simulink library "rewardLibrary"  (R2022b)
settings: Solver=VariableStepAuto  StartTime=0.0  StopTime=10.0  RelTol=1e-3
values from neighbouring files (symbols this model uses):
  accel_vec = (-4:0.5:4)'    [setUpModel.m]
  Ts = 0.1    [setUpMPC.m]
  TsRL = Ts    [setUpRLEnv.m]
  vel_vec = 0:2:20    [setUpModel.m]
undefined symbols (not defined in the file or in its folder): A, B, C, curvature1, D, D_default, DiscIntNeverNeededParam, E, F, gradbp1, k_sigmoid, steer_lim, t_gap, v_set, x_colpen, y_colpen, Z_colpen
libraries: simulink x379, $bdroot x2, mpcadaslib x1
(part 5 of 9)

== system rewardLibrary/Obs // Reward 3-6/Subsystem1 ==
  steer : Inport
  e1 : Inport  Port=2
  v_err : Inport  Port=3
  accel : Inport  Port=4
  Compare To Constant : simulink/Logic and Bit Operations/Compare To Constant  relop=<  const=1  OutDataTypeStr=boolean
  Compare To Constant1 : simulink/Logic and Bit Operations/Compare To Constant  relop=<  const=16  OutDataTypeStr=boolean
  Constant2 : Constant  Value=0
  Constant3 : Constant  Value=5
  Digital Clock : DigitalClock  SampleTime=Ts
  Gain1 : Gain
  Gain2 : Gain  Gain=500
  Gain3 : Gain  Gain=2
  Gain4 : Gain  Gain=1e-3
  Gain6 : Gain  Gain=100
  Gain7 : Gain  Gain=15
  Gain8 : Gain  Gain=100
  Math Function2 : Math  Operator=square  SignedPower=on
  Square : Math  Operator=square  SignedPower=on
  Square2 : Math  Operator=square  SignedPower=on
  Square5 : Math  Operator=square  SignedPower=on
  Sum : Sum  Inputs=-----
  Sum1 : Sum  Inputs=++++
  Switch2 : Switch  Criteria=u2 > Threshold  Threshold=10  SaturateOnIntegerOverflow=off  InputSameDT=off
  Unit Delay : UnitDelay  SampleTime=-1  HasFrameUpgradeWarning=on
  Unit Delay1 : UnitDelay  SampleTime=-1  HasFrameUpgradeWarning=on
  turn assist : Subsystem  Commented=on
  reward : Outport  VectorParamsAs1DForOutWhenUnconnected=off
  wires:
  v_err/1 -> Square5/1
  Square/1 -> Compare To Constant1/1, Gain8/1
  Sum1/1 -> reward/1
  accel/1 -> Unit Delay1/1
  Gain6/1 -> Sum/5
  Compare To Constant/1 -> Gain1/1
  Math Function2/1 -> Gain6/1
  Gain3/1 -> Sum1/1
  Compare To Constant1/1 -> Gain3/1
  Square2/1 -> Gain2/1
  Gain7/1 -> Sum/4
  Unit Delay1/1 -> Math Function2/1
  Gain1/1 -> Sum1/3
  steer/1 -> Unit Delay/1
  Gain2/1 -> Sum/3
  Sum/1 -> Gain4/1
  Unit Delay/1 -> turn assist/1(u_prev), Square2/1  "u_prev"
  Square5/1 -> Compare To Constant/1, Gain7/1
  Gain4/1 -> Sum1/2
  e1/1 -> Square/1
  Digital Clock/1 -> Switch2/2
  Switch2/1 -> Sum1/4
  Gain8/1 -> Sum/1
  Constant2/1 -> Switch2/3
  Constant3/1 -> Switch2/1
  turn assist/1(Out1) -> Sum/2

== system rewardLibrary/Obs // Reward 3-6/Subsystem2 ==
  v_ego : Inport
  e1 : Inport  Port=2
  e2 : Inport  Port=3
  AND : Logic  IconShape=distinctive  AllPortsSameDT=off  OutDataTypeStr=boolean
  Abs : Abs  SaturateOnIntegerOverflow=off
  Abs1 : Abs  SaturateOnIntegerOverflow=off
  Lateral deviation : simulink/Logic and Bit Operations/Compare To Constant  relop=>  const=12  OutDataTypeStr=boolean
  Logical Operator1 : Logic  Operator=OR  AllPortsSameDT=off  OutDataTypeStr=boolean
  R2D : Gain  Gain=180/pi
  Relative yaw angle : simulink/Logic and Bit Operations/Compare To Constant  relop=>  const=55  OutDataTypeStr=boolean
  Velocity : simulink/Logic and Bit Operations/Compare To Constant  relop=<  const=2  OutDataTypeStr=boolean
  Velocity1 : simulink/Logic and Bit Operations/Compare To Constant  relop=<  const=5  OutDataTypeStr=boolean
  offTrack : Outport  VectorParamsAs1DForOutWhenUnconnected=off
  tooSlow / spinTurn : Outport  Port=2  VectorParamsAs1DForOutWhenUnconnected=off
  wires:
  Velocity/1 -> Logical Operator1/1  "tooSlow"
  Lateral deviation/1 -> offTrack/1
  v_ego/1 -> Velocity1/1, Velocity/1
  Abs/1 -> Lateral deviation/1
  e1/1 -> Abs/1
  Velocity1/1 -> AND/1
  e2/1 -> Abs1/1
  Abs1/1 -> R2D/1
  R2D/1 -> Relative yaw angle/1
  Relative yaw angle/1 -> AND/2
  AND/1 -> Logical Operator1/2  "spinTurn"
  Logical Operator1/1 -> tooSlow / spinTurn/1

== system rewardLibrary/Obs // Reward 4-1/Subsystem ==
  v_ego : Inport
  v_ref : Inport  Port=2
  e1 : Inport  Port=3
  e2 : Inport  Port=4
  e1dot : Inport  Port=5
  e2dot : Inport  Port=6
  Add : Sum  Inputs=+-
  Discrete-Time Integrator1 : DiscreteIntegrator  SampleTime=-1  ICPrevOutput=DiscIntNeverNeededParam  ICPrevScaledInput=DiscIntNeverNeededParam
  Discrete-Time Integrator2 : DiscreteIntegrator  SampleTime=-1  ICPrevOutput=DiscIntNeverNeededParam  ICPrevScaledInput=DiscIntNeverNeededParam
  Discrete-Time Integrator3 : DiscreteIntegrator  SampleTime=-1  ICPrevOutput=DiscIntNeverNeededParam  ICPrevScaledInput=DiscIntNeverNeededParam
  Lateral deviation : Scope
  Mux : Mux  Inputs=9
  obs : Outport  VectorParamsAs1DForOutWhenUnconnected=off
  v_err : Outport  Port=2  VectorParamsAs1DForOutWhenUnconnected=off
  wires:
  Add/1 -> v_err/1, Mux/2, Discrete-Time Integrator1/1
  Discrete-Time Integrator3/1 -> Mux/6  "integral_error"
  v_ego/1 -> Add/2, Mux/3
  e1/1 -> Lateral deviation/1, Mux/5, Discrete-Time Integrator2/1
  Discrete-Time Integrator1/1 -> Mux/1  "integral_error"
  e2/1 -> Mux/7, Discrete-Time Integrator3/1
  Discrete-Time Integrator2/1 -> Mux/4  "integral_error"
  Mux/1 -> obs/1
  e1dot/1 -> Mux/8
  e2dot/1 -> Mux/9
  v_ref/1 -> Add/1  "d_rel"

== system rewardLibrary/Obs // Reward 4-1/Subsystem1 ==
  steer : Inport
  e1 : Inport  Port=2
  v_err : Inport  Port=3
  accel : Inport  Port=4
  Compare To Constant : simulink/Logic and Bit Operations/Compare To Constant  relop=<  const=1  OutDataTypeStr=boolean
  Compare To Constant1 : simulink/Logic and Bit Operations/Compare To Constant  relop=<  const=16  OutDataTypeStr=boolean
  Compare To Constant2 : simulink/Logic and Bit Operations/Compare To Constant  relop=>  const=-20  OutDataTypeStr=boolean
  Constant : Constant  Value=1000
  Constant1 : Constant  Value=0
  Demux : Demux  Outputs=2
  Detect Rise Positive : simulink/Logic and Bit Operations/Detect Rise Positive  vinit=0  OutDataTypeStr=boolean
  Gain1 : Gain
  Gain2 : Gain  Gain=500
  Gain3 : Gain  Gain=2
  Gain4 : Gain  Gain=1e-3
  Gain6 : Gain  Gain=100
  Gain7 : Gain  Gain=20
  Gain8 : Gain  Gain=100
  Math Function2 : Math  Operator=square  SignedPower=on
  Square : Math  Operator=square  SignedPower=on
  Square2 : Math  Operator=square  SignedPower=on
  Square5 : Math  Operator=square  SignedPower=on
  Sum : Sum  Inputs=-----
  Sum1 : Sum  Inputs=++++
  Switch : Switch  Criteria=u2 > Threshold  SaturateOnIntegerOverflow=off  InputSameDT=off
  Terminator : Terminator
  Unit Delay : UnitDelay  SampleTime=-1  HasFrameUpgradeWarning=on
  Unit Delay1 : UnitDelay  SampleTime=-1  HasFrameUpgradeWarning=on
  time reward : Subsystem  Commented=on
  turn assist : Subsystem  Commented=on
  reward : Outport  VectorParamsAs1DForOutWhenUnconnected=off
  wires:
  v_err/1 -> Square5/1
  Square/1 -> Compare To Constant1/1, Gain8/1
  Sum1/1 -> reward/1
  accel/1 -> Unit Delay1/1
  Gain6/1 -> Sum/5
  Compare To Constant/1 -> Gain1/1
  Math Function2/1 -> Gain6/1
  Gain3/1 -> Sum1/1
  Compare To Constant1/1 -> Gain3/1
  Square2/1 -> Gain2/1
  Gain7/1 -> Sum/4
  Unit Delay1/1 -> Math Function2/1
  Gain1/1 -> Sum1/3
  steer/1 -> Unit Delay/1
  Gain2/1 -> Sum/3
  Sum/1 -> Gain4/1
  Unit Delay/1 -> turn assist/1(u_prev), Square2/1  "u_prev"
  Square5/1 -> Compare To Constant/1, Gain7/1
  Gain4/1 -> Sum1/2
  e1/1 -> Square/1
  Gain8/1 -> Sum/1
  turn assist/1(Out1) -> Sum/2
  [pos2] -> Demux/1
  Demux/1 -> Terminator/1
  Demux/2 -> Compare To Constant2/1  "y2"
  Constant/1 -> Switch/1
  Constant1/1 -> Switch/3
  Compare To Constant2/1 -> Detect Rise Positive/1
  Detect Rise Positive/1 -> Switch/2
  Switch/1 -> Sum1/4  "madeCorner"

== system rewardLibrary/Obs // Reward 4-1/Subsystem2 ==
  v_ego : Inport
  e1 : Inport  Port=2
  e2 : Inport  Port=3
  AND : Logic  IconShape=distinctive  AllPortsSameDT=off  OutDataTypeStr=boolean
  Abs : Abs  SaturateOnIntegerOverflow=off
  Abs1 : Abs  SaturateOnIntegerOverflow=off
  Lateral deviation : simulink/Logic and Bit Operations/Compare To Constant  relop=>  const=12  OutDataTypeStr=boolean
  Logical Operator1 : Logic  Operator=OR  AllPortsSameDT=off  OutDataTypeStr=boolean
  R2D : Gain  Gain=180/pi
  Relative yaw angle : simulink/Logic and Bit Operations/Compare To Constant  relop=>  const=55  OutDataTypeStr=boolean
  Velocity : simulink/Logic and Bit Operations/Compare To Constant  relop=<  const=2  OutDataTypeStr=boolean
  Velocity1 : simulink/Logic and Bit Operations/Compare To Constant  relop=<  const=5  OutDataTypeStr=boolean
  offTrack : Outport  VectorParamsAs1DForOutWhenUnconnected=off
  tooSlow / spinTurn : Outport  Port=2  VectorParamsAs1DForOutWhenUnconnected=off
  wires:
  Velocity/1 -> Logical Operator1/1  "tooSlow"
  Lateral deviation/1 -> offTrack/1
  v_ego/1 -> Velocity1/1, Velocity/1
  Abs/1 -> Lateral deviation/1
  e1/1 -> Abs/1
  Velocity1/1 -> AND/1
  e2/1 -> Abs1/1
  Abs1/1 -> R2D/1
  R2D/1 -> Relative yaw angle/1
  Relative yaw angle/1 -> AND/2
  AND/1 -> Logical Operator1/2  "spinTurn"
  Logical Operator1/1 -> tooSlow / spinTurn/1

== system rewardLibrary/Obs // Reward 4-2/Subsystem ==
  v_ego : Inport
  v_ref : Inport  Port=2
  e1 : Inport  Port=3
  e2 : Inport  Port=4
  e1dot : Inport  Port=5
  e2dot : Inport  Port=6
  Add : Sum  Inputs=+-
  Discrete-Time Integrator1 : DiscreteIntegrator  SampleTime=-1  ICPrevOutput=DiscIntNeverNeededParam  ICPrevScaledInput=DiscIntNeverNeededParam
  Discrete-Time Integrator2 : DiscreteIntegrator  SampleTime=-1  ICPrevOutput=DiscIntNeverNeededParam  ICPrevScaledInput=DiscIntNeverNeededParam
  Discrete-Time Integrator3 : DiscreteIntegrator  SampleTime=-1  ICPrevOutput=DiscIntNeverNeededParam  ICPrevScaledInput=DiscIntNeverNeededParam
  Lateral deviation : Scope
  Mux : Mux  Inputs=9
  obs : Outport  VectorParamsAs1DForOutWhenUnconnected=off
  v_err : Outport  Port=2  VectorParamsAs1DForOutWhenUnconnected=off
  wires:
  Add/1 -> v_err/1, Mux/2, Discrete-Time Integrator1/1
  Discrete-Time Integrator3/1 -> Mux/6  "integral_error"
  v_ego/1 -> Add/2, Mux/3
  e1/1 -> Lateral deviation/1, Mux/5, Discrete-Time Integrator2/1
  Discrete-Time Integrator1/1 -> Mux/1  "integral_error"
  e2/1 -> Mux/7, Discrete-Time Integrator3/1
  Discrete-Time Integrator2/1 -> Mux/4  "integral_error"
  Mux/1 -> obs/1
  e1dot/1 -> Mux/8
  e2dot/1 -> Mux/9
  v_ref/1 -> Add/1  "d_rel"

== system rewardLibrary/Obs // Reward 4-2/Subsystem1 ==
  steer : Inport
  e1 : Inport  Port=2
  v_err : Inport  Port=3
  accel : Inport  Port=4
  Compare To Constant : simulink/Logic and Bit Operations/Compare To Constant  relop=<  const=1  OutDataTypeStr=boolean
  Compare To Constant1 : simulink/Logic and Bit Operations/Compare To Constant  relop=<  const=16  OutDataTypeStr=boolean
  Compare To Constant2 : simulink/Logic and Bit Operations/Compare To Constant  relop=>  const=-20  OutDataTypeStr=boolean
  Constant : Constant  Value=1000
  Constant1 : Constant  Value=0
  Demux : Demux  Outputs=2
  Detect Rise Positive : simulink/Logic and Bit Operations/Detect Rise Positive  vinit=0  OutDataTypeStr=boolean
  Gain1 : Gain
  Gain2 : Gain  Gain=500
  Gain3 : Gain  Gain=2
  Gain4 : Gain  Gain=1e-3
  Gain6 : Gain  Gain=100
  Gain7 : Gain  Gain=20
  Gain8 : Gain  Gain=100
  Math Function2 : Math  Operator=square  SignedPower=on
  Square : Math  Operator=square  SignedPower=on
  Square2 : Math  Operator=square  SignedPower=on
  Square5 : Math  Operator=square  SignedPower=on
  Sum : Sum  Inputs=-----
  Sum1 : Sum  Inputs=++++
  Switch : Switch  Criteria=u2 > Threshold  SaturateOnIntegerOverflow=off  InputSameDT=off
  Terminator : Terminator
  Unit Delay : UnitDelay  SampleTime=-1  HasFrameUpgradeWarning=on
  Unit Delay1 : UnitDelay  SampleTime=-1  HasFrameUpgradeWarning=on
  time reward : Subsystem  Commented=on
  turn assist : Subsystem  Commented=on
  reward : Outport  VectorParamsAs1DForOutWhenUnconnected=off
  wires:
  v_err/1 -> Square5/1
  Square/1 -> Compare To Constant1/1, Gain8/1
  Sum1/1 -> reward/1
  accel/1 -> Unit Delay1/1
  Gain6/1 -> Sum/5
  Compare To Constant/1 -> Gain1/1
  Math Function2/1 -> Gain6/1
  Gain3/1 -> Sum1/1
  Compare To Constant1/1 -> Gain3/1
  Square2/1 -> Gain2/1
  Gain7/1 -> Sum/4
  Unit Delay1/1 -> Math Function2/1
  Gain1/1 -> Sum1/3
  steer/1 -> Unit Delay/1
  Gain2/1 -> Sum/3
  Sum/1 -> Gain4/1
  Unit Delay/1 -> turn assist/1(u_prev), Square2/1  "u_prev"
  Square5/1 -> Compare To Constant/1, Gain7/1
  Gain4/1 -> Sum1/2
  e1/1 -> Square/1
  Gain8/1 -> Sum/1
  turn assist/1(Out1) -> Sum/2
  [pos2] -> Demux/1
  Demux/1 -> Terminator/1
  Demux/2 -> Compare To Constant2/1  "y2"
  Constant/1 -> Switch/1
  Constant1/1 -> Switch/3
  Compare To Constant2/1 -> Detect Rise Positive/1
  Detect Rise Positive/1 -> Switch/2
  Switch/1 -> Sum1/4  "madeCorner"

== system rewardLibrary/Obs // Reward 4-2/Subsystem2 ==
  v_ego : Inport
  e1 : Inport  Port=2
  e2 : Inport  Port=3
  AND : Logic  IconShape=distinctive  AllPortsSameDT=off  OutDataTypeStr=boolean
  Abs : Abs  SaturateOnIntegerOverflow=off
  Abs1 : Abs  SaturateOnIntegerOverflow=off
  Lateral deviation : simulink/Logic and Bit Operations/Compare To Constant  relop=>  const=8  OutDataTypeStr=boolean
  R2D : Gain  Gain=180/pi
  Relative yaw angle : simulink/Logic and Bit Operations/Compare To Constant  relop=>  const=55  OutDataTypeStr=boolean
  Velocity : simulink/Logic and Bit Operations/Compare To Constant  relop=<  const=2  OutDataTypeStr=boolean
  Velocity1 : simulink/Logic and Bit Operations/Compare To Constant  relop=<  const=5  OutDataTypeStr=boolean
  offTrack : Outport  VectorParamsAs1DForOutWhenUnconnected=off
  tooSlow : Outport  Port=2  VectorParamsAs1DForOutWhenUnconnected=off
  spinTurn : Outport  Port=3  VectorParamsAs1DForOutWhenUnconnected=off
  wires:
  Velocity/1 -> tooSlow/1  "tooSlow"
  Lateral deviation/1 -> offTrack/1
  v_ego/1 -> Velocity1/1, Velocity/1
  Abs/1 -> Lateral deviation/1
  e1/1 -> Abs/1
  Velocity1/1 -> AND/1
  e2/1 -> Abs1/1
  Abs1/1 -> R2D/1
  R2D/1 -> Relative yaw angle/1
  Relative yaw angle/1 -> AND/2
  AND/1 -> spinTurn/1  "spinTurn"

== system rewardLibrary/Obs // Reward 5-1/Subsystem ==
  v_ego : Inport
  v_ref : Inport  Port=2
  e1 : Inport  Port=3
  e2 : Inport  Port=4
  e1dot : Inport  Port=5
  e2dot : Inport  Port=6
  Add : Sum  Inputs=+-
  Discrete-Time Integrator1 : DiscreteIntegrator  SampleTime=-1  ICPrevOutput=DiscIntNeverNeededParam  ICPrevScaledInput=DiscIntNeverNeededParam
  Discrete-Time Integrator2 : DiscreteIntegrator  SampleTime=-1  ICPrevOutput=DiscIntNeverNeededParam  ICPrevScaledInput=DiscIntNeverNeededParam
  Discrete-Time Integrator3 : DiscreteIntegrator  SampleTime=-1  ICPrevOutput=DiscIntNeverNeededParam  ICPrevScaledInput=DiscIntNeverNeededParam
  Lateral deviation : Scope
  Mux : Mux  Inputs=9
  obs : Outport  VectorParamsAs1DForOutWhenUnconnected=off
  v_err : Outport  Port=2  VectorParamsAs1DForOutWhenUnconnected=off
  wires:
  Add/1 -> v_err/1, Mux/2, Discrete-Time Integrator1/1
  Discrete-Time Integrator3/1 -> Mux/6  "integral_error"
  v_ego/1 -> Add/2, Mux/3
  e1/1 -> Lateral deviation/1, Mux/5, Discrete-Time Integrator2/1
  Discrete-Time Integrator1/1 -> Mux/1  "integral_error"
  e2/1 -> Mux/7, Discrete-Time Integrator3/1
  Discrete-Time Integrator2/1 -> Mux/4  "integral_error"
  Mux/1 -> obs/1
  e1dot/1 -> Mux/8
  e2dot/1 -> Mux/9
  v_ref/1 -> Add/1  "d_rel"

== system rewardLibrary/Obs // Reward 5-1/Subsystem1 ==
  v_err : Inport
  e1 : Inport  Port=2
  e2 : Inport  Port=3
  steer : Inport  Port=4
  accel : Inport  Port=5
  Exp{,1..4} (5 alike) : Math
  Gain1 : Gain  Gain=0.5
  Gain10 : Gain  Gain=-0.1
  Gain2 : Gain  Gain=0.2
  Gain3 : Gain  Gain=0.1
  Gain4 : Gain  Gain=-0.5
  Gain5 : Gain  Gain=-10
  Gain6 : Gain  Gain=1.5
  Gain7 : Gain
  Gain8 : Gain  Gain=-0.1
  Gain9 : Gain  Gain=-1.5
  Math Function2 : Math  Operator=square  SignedPower=on
  Square{1..3,5} (4 alike) : Math  Operator=square  SignedPower=on
  Sum1 : Sum  Inputs=+++++
  Unit Delay : UnitDelay  SampleTime=-1  HasFrameUpgradeWarning=on
  Unit Delay1 : UnitDelay  SampleTime=-1  HasFrameUpgradeWarning=on
  reward : Outport  VectorParamsAs1DForOutWhenUnconnected=off
  wires:
  Sum1/1 -> reward/1
  accel/1 -> Unit Delay1/1
  Square2/1 -> Gain4/1
  steer/1 -> Unit Delay/1
  Square5/1 -> Gain10/1
  e1/1 -> Square1/1
  v_err/1 -> Square5/1
  e2/1 -> Square2/1
  Unit Delay/1 -> Math Function2/1  "u_prev"
  Unit Delay1/1 -> Square3/1
  Square3/1 -> Gain8/1
  Math Function2/1 -> Gain5/1
  Square1/1 -> Gain9/1
  Gain10/1 -> Exp/1
  Gain8/1 -> Exp4/1
  Gain5/1 -> Exp3/1
  Gain4/1 -> Exp2/1
  Gain9/1 -> Exp1/1
  Exp/1 -> Gain7/1
  Exp1/1 -> Gain6/1
  Exp2/1 -> Gain1/1
  Exp3/1 -> Gain2/1
  Exp4/1 -> Gain3/1
  Gain3/1 -> Sum1/5
  Gain2/1 -> Sum1/4
  Gain1/1 -> Sum1/3
  Gain6/1 -> Sum1/2
  Gain7/1 -> Sum1/1

== system rewardLibrary/Obs // Reward 5-1/Subsystem2 ==
  v_ego : Inport
  e1 : Inport  Port=2
  e2 : Inport  Port=3
  AND : Logic  Commented=on  IconShape=distinctive  AllPortsSameDT=off  OutDataTypeStr=boolean
  Abs : Abs  SaturateOnIntegerOverflow=off
  Abs1 : Abs  Commented=on  SaturateOnIntegerOverflow=off
  Lateral deviation : simulink/Logic and Bit Operations/Compare To Constant  relop=>  const=8  OutDataTypeStr=boolean
  R2D : Gain  Commented=on  Gain=180/pi
  Relative yaw angle : simulink/Logic and Bit Operations/Compare To Constant  Commented=on  relop=>  const=55  OutDataTypeStr=boolean
  Velocity : simulink/Logic and Bit Operations/Compare To Constant  relop=<  const=2  OutDataTypeStr=boolean
  Velocity1 : simulink/Logic and Bit Operations/Compare To Constant  Commented=on  relop=<  const=5  OutDataTypeStr=boolean
  offTrack : Outport  VectorParamsAs1DForOutWhenUnconnected=off
  tooSlow : Outport  Port=2  VectorParamsAs1DForOutWhenUnconnected=off
  spinTurn : Outport  Port=3  VectorParamsAs1DForOutWhenUnconnected=off
  wires:
  Velocity/1 -> tooSlow/1  "tooSlow"
  Lateral deviation/1 -> offTrack/1
  v_ego/1 -> Velocity1/1, Velocity/1
  Abs/1 -> Lateral deviation/1
  e1/1 -> Abs/1
  Velocity1/1 -> AND/1
  e2/1 -> Abs1/1
  Abs1/1 -> R2D/1
  R2D/1 -> Relative yaw angle/1
  Relative yaw angle/1 -> AND/2
  AND/1 -> spinTurn/1  "spinTurn"

== system rewardLibrary/Obs // Reward 5-2/Subsystem ==
  v_ego : Inport
  v_ref : Inport  Port=2
  e1 : Inport  Port=3
  e2 : Inport  Port=4
  e1dot : Inport  Port=5
  e2dot : Inport  Port=6
  Add : Sum  Inputs=+-
  Discrete-Time Integrator1 : DiscreteIntegrator  SampleTime=-1  ICPrevOutput=DiscIntNeverNeededParam  ICPrevScaledInput=DiscIntNeverNeededParam
  Discrete-Time Integrator2 : DiscreteIntegrator  SampleTime=-1  ICPrevOutput=DiscIntNeverNeededParam  ICPrevScaledInput=DiscIntNeverNeededParam
  Discrete-Time Integrator3 : DiscreteIntegrator  SampleTime=-1  ICPrevOutput=DiscIntNeverNeededParam  ICPrevScaledInput=DiscIntNeverNeededParam
  Lateral deviation : Scope
  Mux : Mux  Inputs=9
  obs : Outport  VectorParamsAs1DForOutWhenUnconnected=off
  v_err : Outport  Port=2  VectorParamsAs1DForOutWhenUnconnected=off
  wires:
  Add/1 -> v_err/1, Mux/2, Discrete-Time Integrator1/1
  Discrete-Time Integrator3/1 -> Mux/6  "integral_error"
  v_ego/1 -> Add/2, Mux/3
  e1/1 -> Lateral deviation/1, Mux/5, Discrete-Time Integrator2/1
  Discrete-Time Integrator1/1 -> Mux/1  "integral_error"
  e2/1 -> Mux/7, Discrete-Time Integrator3/1
  Discrete-Time Integrator2/1 -> Mux/4  "integral_error"
  Mux/1 -> obs/1
  e1dot/1 -> Mux/8
  e2dot/1 -> Mux/9
  v_ref/1 -> Add/1  "d_rel"

== system rewardLibrary/Obs // Reward 5-2/Subsystem1 ==
  v_err : Inport
  e1 : Inport  Port=2
  e2 : Inport  Port=3
  steer : Inport  Port=4
  accel : Inport  Port=5
  Exp{,1..4} (5 alike) : Math
  Gain1 : Gain  Gain=0.5
  Gain10 : Gain  Gain=-0.1
  Gain2 : Gain  Gain=0.2
  Gain3 : Gain  Gain=0.1
  Gain4 : Gain  Gain=-0.5
  Gain5 : Gain  Gain=-10
  Gain6 : Gain  Gain=1.5
  Gain7 : Gain
  Gain8 : Gain  Gain=-0.1
  Gain9 : Gain  Gain=-1.5
  Math Function2 : Math  Operator=square  SignedPower=on
  Square{1..3,5} (4 alike) : Math  Operator=square  SignedPower=on
  Sum1 : Sum  Inputs=+++++
  Unit Delay : UnitDelay  SampleTime=-1  HasFrameUpgradeWarning=on
  Unit Delay1 : UnitDelay  SampleTime=-1  HasFrameUpgradeWarning=on
  reward : Outport  VectorParamsAs1DForOutWhenUnconnected=off
  wires:
  Sum1/1 -> reward/1
  accel/1 -> Unit Delay1/1
  Square2/1 -> Gain4/1
  steer/1 -> Unit Delay/1
  Square5/1 -> Gain10/1
  e1/1 -> Square1/1
  v_err/1 -> Square5/1
  e2/1 -> Square2/1
  Unit Delay/1 -> Math Function2/1  "u_prev"
  Unit Delay1/1 -> Square3/1
  Square3/1 -> Gain8/1
  Math Function2/1 -> Gain5/1
  Square1/1 -> Gain9/1
  Gain10/1 -> Exp/1
  Gain8/1 -> Exp4/1
  Gain5/1 -> Exp3/1
  Gain4/1 -> Exp2/1
  Gain9/1 -> Exp1/1
  Exp/1 -> Gain7/1
  Exp1/1 -> Gain6/1
  Exp2/1 -> Gain1/1
  Exp3/1 -> Gain2/1
  Exp4/1 -> Gain3/1
  Gain3/1 -> Sum1/5
  Gain2/1 -> Sum1/4
  Gain1/1 -> Sum1/3
  Gain6/1 -> Sum1/2
  Gain7/1 -> Sum1/1

== system rewardLibrary/Obs // Reward 5-2/Subsystem2 ==
  v_ego : Inport
  e1 : Inport  Port=2
  e2 : Inport  Port=3
  AND : Logic  IconShape=distinctive  AllPortsSameDT=off  OutDataTypeStr=boolean
  Abs : Abs  SaturateOnIntegerOverflow=off
  Abs1 : Abs  SaturateOnIntegerOverflow=off
  Lateral deviation : simulink/Logic and Bit Operations/Compare To Constant  relop=>  const=8  OutDataTypeStr=boolean
  R2D : Gain  Gain=180/pi
  Relative yaw angle : simulink/Logic and Bit Operations/Compare To Constant  relop=>  const=55  OutDataTypeStr=boolean
  Velocity : simulink/Logic and Bit Operations/Compare To Constant  relop=<  const=2  OutDataTypeStr=boolean
  Velocity1 : simulink/Logic and Bit Operations/Compare To Constant  relop=<  const=5  OutDataTypeStr=boolean
  offTrack : Outport  VectorParamsAs1DForOutWhenUnconnected=off
  tooSlow : Outport  Port=2  VectorParamsAs1DForOutWhenUnconnected=off
  spinTurn : Outport  Port=3  VectorParamsAs1DForOutWhenUnconnected=off
  wires:
  Velocity/1 -> tooSlow/1  "tooSlow"
  Lateral deviation/1 -> offTrack/1
  v_ego/1 -> Velocity1/1, Velocity/1
  Abs/1 -> Lateral deviation/1
  e1/1 -> Abs/1
  Velocity1/1 -> AND/1
  e2/1 -> Abs1/1
  Abs1/1 -> R2D/1
  R2D/1 -> Relative yaw angle/1
  Relative yaw angle/1 -> AND/2
  AND/1 -> spinTurn/1  "spinTurn"

== system rewardLibrary/Obs // Reward 5-3/Subsystem ==
  v_ego : Inport
  v_ref : Inport  Port=2
  e1 : Inport  Port=3
  e2 : Inport  Port=4
  e1dot : Inport  Port=5
  e2dot : Inport  Port=6
  Add : Sum  Inputs=+-
  Discrete-Time Integrator1 : DiscreteIntegrator  SampleTime=-1  ICPrevOutput=DiscIntNeverNeededParam  ICPrevScaledInput=DiscIntNeverNeededParam
  Discrete-Time Integrator2 : DiscreteIntegrator  SampleTime=-1  ICPrevOutput=DiscIntNeverNeededParam  ICPrevScaledInput=DiscIntNeverNeededParam
  Discrete-Time Integrator3 : DiscreteIntegrator  SampleTime=-1  ICPrevOutput=DiscIntNeverNeededParam  ICPrevScaledInput=DiscIntNeverNeededParam
  Lateral deviation : Scope
  Mux : Mux  Inputs=9
  obs : Outport  VectorParamsAs1DForOutWhenUnconnected=off
  v_err : Outport  Port=2  VectorParamsAs1DForOutWhenUnconnected=off
  wires:
  Add/1 -> v_err/1, Mux/2, Discrete-Time Integrator1/1
  Discrete-Time Integrator3/1 -> Mux/6  "integral_error"
  v_ego/1 -> Add/2, Mux/3
  e1/1 -> Lateral deviation/1, Mux/5, Discrete-Time Integrator2/1
  Discrete-Time Integrator1/1 -> Mux/1  "integral_error"
  e2/1 -> Mux/7, Discrete-Time Integrator3/1
  Discrete-Time Integrator2/1 -> Mux/4  "integral_error"
  Mux/1 -> obs/1
  e1dot/1 -> Mux/8
  e2dot/1 -> Mux/9
  v_ref/1 -> Add/1  "d_rel"

== system rewardLibrary/Obs // Reward 5-3/Subsystem1 ==
  v_err : Inport
  e1 : Inport  Port=2
  e2 : Inport  Port=3
  steer : Inport  Port=4
  accel : Inport  Port=5
  Add : Sum  Inputs=+-
  Constant : Constant
  Exp{1..4} (4 alike) : Math
  Gain1 : Gain  Gain=0.5
  Gain10 : Gain  Gain=0.1
  Gain2 : Gain  Gain=0.2
  Gain3 : Gain  Gain=0.1
  Gain4 : Gain  Gain=-0.5
  Gain5 : Gain  Gain=-10
  Gain6 : Gain  Gain=1.5
  Gain7 : Gain  Gain=0.05
  Gain8 : Gain  Gain=-0.1
  Gain9 : Gain  Gain=-1.5
  Math Function2 : Math  Operator=square  SignedPower=on
  Square{1..3,5} (4 alike) : Math  Operator=square  SignedPower=on
  Sum1 : Sum  Inputs=+++++
  Unit Delay : UnitDelay  SampleTime=-1  HasFrameUpgradeWarning=on
  Unit Delay1 : UnitDelay  SampleTime=-1  HasFrameUpgradeWarning=on
  reward : Outport  VectorParamsAs1DForOutWhenUnconnected=off
  wires:
  Sum1/1 -> reward/1
  accel/1 -> Unit Delay1/1
  Square2/1 -> Gain4/1
  steer/1 -> Unit Delay/1
  Square5/1 -> Gain10/1
  e1/1 -> Square1/1
  v_err/1 -> Square5/1
  e2/1 -> Square2/1
  Unit Delay/1 -> Math Function2/1  "u_prev"
  Unit Delay1/1 -> Square3/1
  Square3/1 -> Gain8/1
  Math Function2/1 -> Gain5/1
  Square1/1 -> Gain9/1
  Gain8/1 -> Exp4/1
  Gain5/1 -> Exp3/1
  Gain4/1 -> Exp2/1
  Gain9/1 -> Exp1/1
  Add/1 -> Gain7/1
  Exp1/1 -> Gain6/1
  Exp2/1 -> Gain1/1
  Exp3/1 -> Gain2/1
  Exp4/1 -> Gain3/1
  Gain3/1 -> Sum1/5
  Gain2/1 -> Sum1/4
  Gain1/1 -> Sum1/3
  Gain6/1 -> Sum1/2
  Gain7/1 -> Sum1/1
  Constant/1 -> Add/1
  Gain10/1 -> Add/2

== system rewardLibrary/Obs // Reward 5-3/Subsystem2 ==
  v_ego : Inport
  e1 : Inport  Port=2
  e2 : Inport  Port=3
  AND : Logic  IconShape=distinctive  AllPortsSameDT=off  OutDataTypeStr=boolean
  Abs : Abs  SaturateOnIntegerOverflow=off
  Abs1 : Abs  SaturateOnIntegerOverflow=off
  Constant : Constant
  Constant3 : Constant  Value=0
  Demux : Demux  Outputs=2
  Lateral deviation : simulink/Logic and Bit Operations/Compare To Constant  relop=>  const=8  OutDataTypeStr=boolean
  Logical Operator1 : Logic  Operator=OR  Inputs=3  AllPortsSameDT=off  OutDataTypeStr=boolean
  R2D : Gain  Gain=180/pi
  Relative yaw angle : simulink/Logic and Bit Operations/Compare To Constant  relop=>  const=60  OutDataTypeStr=boolean
  Switch : Switch  Criteria=u2 > Threshold  Threshold=90  SaturateOnIntegerOverflow=off  InputSameDT=off
  Terminator : Terminator
  Velocity : simulink/Logic and Bit Operations/Compare To Constant  relop=<  const=2  OutDataTypeStr=boolean
  Velocity1 : simulink/Logic and Bit Operations/Compare To Constant  relop=<  const=10  OutDataTypeStr=boolean
  fail : Outport  VectorParamsAs1DForOutWhenUnconnected=off
  success : Outport  Port=2  VectorParamsAs1DForOutWhenUnconnected=off
  wires:
  Velocity/1 -> Logical Operator1/1  "tooSlow"
  Lateral deviation/1 -> Logical Operator1/2
  v_ego/1 -> Velocity1/1, Velocity/1
  Abs/1 -> Lateral deviation/1
  e1/1 -> Abs/1
  Velocity1/1 -> AND/1
  e2/1 -> Abs1/1
  Abs1/1 -> R2D/1
  R2D/1 -> Relative yaw angle/1
  Relative yaw angle/1 -> AND/2
  AND/1 -> Logical Operator1/3  "spinTurn"
  Switch/1 -> success/1
  Constant/1 -> Switch/1
  Constant3/1 -> Switch/3
  Logical Operator1/1 -> fail/1
  Demux/1 -> Terminator/1
  [pos2] -> Demux/1
  Demux/2 -> Switch/2  "y2"

== system rewardLibrary/Obs // Reward 5-4/Subsystem ==
  v_ego : Inport
  v_ref : Inport  Port=2
  e1 : Inport  Port=3
  e2 : Inport  Port=4
  e1dot : Inport  Port=5
  e2dot : Inport  Port=6
  Add : Sum  Inputs=+-
  Discrete-Time Integrator1 : DiscreteIntegrator  SampleTime=-1  ICPrevOutput=DiscIntNeverNeededParam  ICPrevScaledInput=DiscIntNeverNeededParam
  Discrete-Time Integrator2 : DiscreteIntegrator  SampleTime=-1  ICPrevOutput=DiscIntNeverNeededParam  ICPrevScaledInput=DiscIntNeverNeededParam
  Discrete-Time Integrator3 : DiscreteIntegrator  SampleTime=-1  ICPrevOutput=DiscIntNeverNeededParam  ICPrevScaledInput=DiscIntNeverNeededParam
  Lateral deviation : Scope
  Mux : Mux  Inputs=9
  obs : Outport  VectorParamsAs1DForOutWhenUnconnected=off
  v_err : Outport  Port=2  VectorParamsAs1DForOutWhenUnconnected=off
  wires:
  Add/1 -> v_err/1, Mux/2, Discrete-Time Integrator1/1
  Discrete-Time Integrator3/1 -> Mux/6  "integral_error"
  v_ego/1 -> Add/2, Mux/3
  e1/1 -> Lateral deviation/1, Mux/5, Discrete-Time Integrator2/1
  Discrete-Time Integrator1/1 -> Mux/1  "integral_error"
  e2/1 -> Mux/7, Discrete-Time Integrator3/1
  Discrete-Time Integrator2/1 -> Mux/4  "integral_error"
  Mux/1 -> obs/1
  e1dot/1 -> Mux/8
  e2dot/1 -> Mux/9
  v_ref/1 -> Add/1  "d_rel"

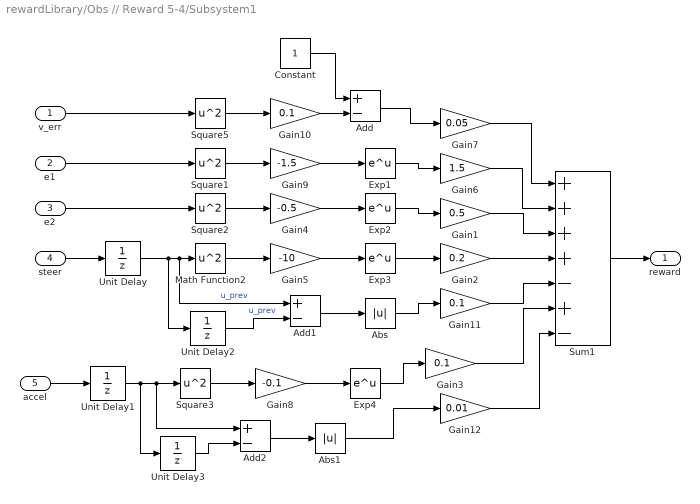
== system rewardLibrary/Obs // Reward 5-4/Subsystem1 ==
  v_err : Inport
  e1 : Inport  Port=2
  e2 : Inport  Port=3
  steer : Inport  Port=4
  accel : Inport  Port=5
  Abs : Abs  SaturateOnIntegerOverflow=off
  Abs1 : Abs  SaturateOnIntegerOverflow=off
  Add : Sum  Inputs=+-
  Add1 : Sum  Inputs=+-
  Add2 : Sum  Inputs=+-
  Constant : Constant
  Exp{1..4} (4 alike) : Math
  Gain1 : Gain  Gain=0.5
  Gain10 : Gain  Gain=0.1
  Gain11 : Gain  Gain=0.1
  Gain12 : Gain  Gain=0.01
  Gain2 : Gain  Gain=0.2
  Gain3 : Gain  Gain=0.1
  Gain4 : Gain  Gain=-0.5
  Gain5 : Gain  Gain=-10
  Gain6 : Gain  Gain=1.5
  Gain7 : Gain  Gain=0.05
  Gain8 : Gain  Gain=-0.1
  Gain9 : Gain  Gain=-1.5
  Math Function2 : Math  Operator=square  SignedPower=on
  Square{1..3,5} (4 alike) : Math  Operator=square  SignedPower=on
  Sum1 : Sum  Inputs=++++-+-
  Unit Delay{,1..3} (4 alike) : UnitDelay  SampleTime=-1  HasFrameUpgradeWarning=on
  reward : Outport  VectorParamsAs1DForOutWhenUnconnected=off
  wires:
  Sum1/1 -> reward/1
  accel/1 -> Unit Delay1/1
  Square2/1 -> Gain4/1
  steer/1 -> Unit Delay/1
  Square5/1 -> Gain10/1
  e1/1 -> Square1/1
  v_err/1 -> Square5/1
  e2/1 -> Square2/1
  Unit Delay/1 -> Unit Delay2/1, Add1/1, Math Function2/1  "u_prev"
  Unit Delay1/1 -> Unit Delay3/1, Add2/1, Square3/1
  Square3/1 -> Gain8/1
  Math Function2/1 -> Gain5/1
  Square1/1 -> Gain9/1
  Gain8/1 -> Exp4/1
  Gain5/1 -> Exp3/1
  Gain4/1 -> Exp2/1
  Gain9/1 -> Exp1/1
  Add/1 -> Gain7/1
  Exp1/1 -> Gain6/1
  Exp2/1 -> Gain1/1
  Exp3/1 -> Gain2/1
  Exp4/1 -> Gain3/1
  Gain3/1 -> Sum1/6
  Gain2/1 -> Sum1/4
  Gain1/1 -> Sum1/3
  Gain6/1 -> Sum1/2
  Gain7/1 -> Sum1/1
  Constant/1 -> Add/1
  Gain10/1 -> Add/2
  Unit Delay2/1 -> Add1/2  "u_prev"
  Add1/1 -> Abs/1
  Gain11/1 -> Sum1/5
  Abs/1 -> Gain11/1
  Unit Delay3/1 -> Add2/2
  Add2/1 -> Abs1/1
  Abs1/1 -> Gain12/1
  Gain12/1 -> Sum1/7

== system rewardLibrary/Obs // Reward 5-4/Subsystem2 ==
  v_ego : Inport
  e1 : Inport  Port=2
  e2 : Inport  Port=3
  AND : Logic  IconShape=distinctive  AllPortsSameDT=off  OutDataTypeStr=boolean
  Abs : Abs  SaturateOnIntegerOverflow=off
  Abs1 : Abs  SaturateOnIntegerOverflow=off
  Constant : Constant
  Constant3 : Constant  Value=0
  Demux : Demux  Outputs=2
  Lateral deviation : simulink/Logic and Bit Operations/Compare To Constant  relop=>  const=8  OutDataTypeStr=boolean
  Logical Operator1 : Logic  Operator=OR  Inputs=3  AllPortsSameDT=off  OutDataTypeStr=boolean
  R2D : Gain  Gain=180/pi
  Relative yaw angle : simulink/Logic and Bit Operations/Compare To Constant  relop=>  const=60  OutDataTypeStr=boolean
  Switch : Switch  Criteria=u2 > Threshold  Threshold=90  SaturateOnIntegerOverflow=off  InputSameDT=off
  Terminator : Terminator
  Velocity : simulink/Logic and Bit Operations/Compare To Constant  relop=<  const=2  OutDataTypeStr=boolean
  Velocity1 : simulink/Logic and Bit Operations/Compare To Constant  relop=<  const=10  OutDataTypeStr=boolean
  fail : Outport  VectorParamsAs1DForOutWhenUnconnected=off
  success : Outport  Port=2  VectorParamsAs1DForOutWhenUnconnected=off
  wires:
  Velocity/1 -> Logical Operator1/1  "tooSlow"
  Lateral deviation/1 -> Logical Operator1/2
  v_ego/1 -> Velocity1/1, Velocity/1
  Abs/1 -> Lateral deviation/1
  e1/1 -> Abs/1
  Velocity1/1 -> AND/1
  e2/1 -> Abs1/1
  Abs1/1 -> R2D/1
  R2D/1 -> Relative yaw angle/1
  Relative yaw angle/1 -> AND/2
  AND/1 -> Logical Operator1/3  "spinTurn"
  Switch/1 -> success/1
  Constant/1 -> Switch/1
  Constant3/1 -> Switch/3
  Logical Operator1/1 -> fail/1
  Demux/1 -> Terminator/1
  [pos2] -> Demux/1
  Demux/2 -> Switch/2  "y2"

== system rewardLibrary/Obs // Reward 6-1/Subsystem ==
  v_ego : Inport
  v_ref : Inport  Port=2
  e1 : Inport  Port=3
  e2 : Inport  Port=4
  e1dot : Inport  Port=5
  e2dot : Inport  Port=6
  v_lead : Inport  Port=7
  xgap : Inport  Port=8
  ygap : Inport  Port=9
  Add : Sum  Inputs=+-
  Discrete-Time Integrator1 : DiscreteIntegrator  SampleTime=-1  ICPrevOutput=DiscIntNeverNeededParam  ICPrevScaledInput=DiscIntNeverNeededParam
  Discrete-Time Integrator2 : DiscreteIntegrator  SampleTime=-1  ICPrevOutput=DiscIntNeverNeededParam  ICPrevScaledInput=DiscIntNeverNeededParam
  Discrete-Time Integrator3 : DiscreteIntegrator  SampleTime=-1  ICPrevOutput=DiscIntNeverNeededParam  ICPrevScaledInput=DiscIntNeverNeededParam
  Lateral deviation : Scope
  Mux : Mux  Inputs=12
  obs : Outport  VectorParamsAs1DForOutWhenUnconnected=off
  v_err : Outport  Port=2  VectorParamsAs1DForOutWhenUnconnected=off
  wires:
  v_ref/1 -> Add/1  "d_rel"
  e2dot/1 -> Mux/9
  e1dot/1 -> Mux/8
  Mux/1 -> obs/1
  Discrete-Time Integrator2/1 -> Mux/4  "integral_error"
  e2/1 -> Discrete-Time Integrator3/1, Mux/7
  Discrete-Time Integrator1/1 -> Mux/1  "integral_error"
  e1/1 -> Discrete-Time Integrator2/1, Mux/5, Lateral deviation/1
  v_ego/1 -> Mux/3, Add/2
  Discrete-Time Integrator3/1 -> Mux/6  "integral_error"
  Add/1 -> Discrete-Time Integrator1/1, Mux/2, v_err/1
  v_lead/1 -> Mux/10
  xgap/1 -> Mux/11
  ygap/1 -> Mux/12

== system rewardLibrary/Obs // Reward 6-1/Subsystem1 ==
  v_err : Inport
  e1 : Inport  Port=2
  e2 : Inport  Port=3
  steer : Inport  Port=4
  accel : Inport  Port=5
  Add : Sum  Inputs=+-
  Constant : Constant
  Exp{1..4} (4 alike) : Math
  Gain1 : Gain  Gain=0.5
  Gain10 : Gain  Gain=0.1
  Gain2 : Gain  Gain=0.2
  Gain3 : Gain  Gain=0.1
  Gain4 : Gain  Gain=-0.5
  Gain5 : Gain  Gain=-10
  Gain6 : Gain  Gain=1.5
  Gain7 : Gain  Gain=0.05
  Gain8 : Gain  Gain=-0.1
  Gain9 : Gain  Gain=-1.5
  Math Function2 : Math  Operator=square  SignedPower=on
  Square{1..3,5} (4 alike) : Math  Operator=square  SignedPower=on
  Sum1 : Sum  Inputs=+++++
  Unit Delay : UnitDelay  SampleTime=-1  HasFrameUpgradeWarning=on
  Unit Delay1 : UnitDelay  SampleTime=-1  HasFrameUpgradeWarning=on
  reward : Outport  VectorParamsAs1DForOutWhenUnconnected=off
  wires:
  Gain10/1 -> Add/2
  Constant/1 -> Add/1
  Gain7/1 -> Sum1/1
  Gain6/1 -> Sum1/2
  Gain1/1 -> Sum1/3
  Gain2/1 -> Sum1/4
  Gain3/1 -> Sum1/5
  Exp4/1 -> Gain3/1
  Exp3/1 -> Gain2/1
  Exp2/1 -> Gain1/1
  Exp1/1 -> Gain6/1
  Add/1 -> Gain7/1
  Gain9/1 -> Exp1/1
  Gain4/1 -> Exp2/1
  Gain5/1 -> Exp3/1
  Gain8/1 -> Exp4/1
  Square1/1 -> Gain9/1
  Math Function2/1 -> Gain5/1
  Square3/1 -> Gain8/1
  Unit Delay1/1 -> Square3/1
  Unit Delay/1 -> Math Function2/1  "u_prev"
  e2/1 -> Square2/1
  v_err/1 -> Square5/1
  e1/1 -> Square1/1
  Square5/1 -> Gain10/1
  steer/1 -> Unit Delay/1
  Square2/1 -> Gain4/1
  accel/1 -> Unit Delay1/1
  Sum1/1 -> reward/1

== system rewardLibrary/Obs // Reward 6-1/Subsystem2 ==
  v_ego : Inport
  e1 : Inport  Port=2
  e2 : Inport  Port=3
  AND : Logic  IconShape=distinctive  AllPortsSameDT=off  OutDataTypeStr=boolean
  Abs : Abs  SaturateOnIntegerOverflow=off
  Abs1 : Abs  SaturateOnIntegerOverflow=off
  Constant : Constant
  Constant3 : Constant  Value=0
  Demux : Demux  Outputs=2
  Lateral deviation : simulink/Logic and Bit Operations/Compare To Constant  relop=>  const=8  OutDataTypeStr=boolean
  Logical Operator1 : Logic  Operator=OR  Inputs=3  AllPortsSameDT=off  OutDataTypeStr=boolean
  R2D : Gain  Gain=180/pi
  Relative yaw angle : simulink/Logic and Bit Operations/Compare To Constant  relop=>  const=60  OutDataTypeStr=boolean
  Switch : Switch  Criteria=u2 > Threshold  Threshold=90  SaturateOnIntegerOverflow=off  InputSameDT=off
  Terminator : Terminator
  Velocity : simulink/Logic and Bit Operations/Compare To Constant  relop=<  const=2  OutDataTypeStr=boolean
  Velocity1 : simulink/Logic and Bit Operations/Compare To Constant  relop=<  const=10  OutDataTypeStr=boolean
  fail : Outport  VectorParamsAs1DForOutWhenUnconnected=off
  success : Outport  Port=2  VectorParamsAs1DForOutWhenUnconnected=off
  wires:
  Demux/2 -> Switch/2  "y2"
  [pos2] -> Demux/1
  Demux/1 -> Terminator/1
  Logical Operator1/1 -> fail/1
  Constant3/1 -> Switch/3
  Constant/1 -> Switch/1
  Switch/1 -> success/1
  AND/1 -> Logical Operator1/3  "spinTurn"
  Relative yaw angle/1 -> AND/2
  R2D/1 -> Relative yaw angle/1
  Abs1/1 -> R2D/1
  e2/1 -> Abs1/1
  Velocity1/1 -> AND/1
  e1/1 -> Abs/1
  Abs/1 -> Lateral deviation/1
  v_ego/1 -> Velocity/1, Velocity1/1
  Lateral deviation/1 -> Logical Operator1/2
  Velocity/1 -> Logical Operator1/1  "tooSlow"

== system rewardLibrary/Obs // Reward 6-2/Overtaking ==
  ry : Inport
  G : Inport  Port=2
  Add : Sum  Inputs=+-
  Compare To Constant : simulink/Logic and Bit Operations/Compare To Constant  Commented=on  relop=>  const=0  OutDataTypeStr=boolean
  Constant : Constant
  Constant1 : Constant  Value=0
  D : Gain  Gain=2
  F : Gain  Commented=on  Gain=3
  Gain1 : Gain  Gain=2
  Gain6 : Gain  Gain=0.75
  Sigmoid : Subsystem
  Slipstream reward enable : Switch  Criteria=u2 > Threshold  Threshold=-5  SaturateOnIntegerOverflow=off  InputSameDT=off
  Sum1 : Sum  Inputs=+++
  r_ot : Outport  VectorParamsAs1DForOutWhenUnconnected=off
  wires:
  Sum1/1 -> r_ot/1
  Slipstream reward enable/1 -> Sum1/1
  ry/1 -> Gain6/1
  Sigmoid/1(sigmoid) -> Gain1/1
  Gain1/1 -> Add/1
  Constant/1 -> Add/2
  D/1 -> Sum1/2
  Add/1 -> D/1
  G/1 -> Compare To Constant/1, Slipstream reward enable/2, Sigmoid/1(x)
  Gain6/1 -> Slipstream reward enable/3
  Constant1/1 -> Slipstream reward enable/1
  F/1 -> Sum1/3
  Compare To Constant/1 -> F/1

== system rewardLibrary/Obs // Reward 6-2/Path following ==
  v_err : Inport
  e1 : Inport  Port=2
  e2 : Inport  Port=3
  steer : Inport  Port=4
  accel : Inport  Port=5
  Exp{,1..4} (5 alike) : Math
  Gain1 : Gain  Gain=0.5
  Gain11 : Gain  Gain=-0.1
  Gain12 : Gain  Gain=1.5
  Gain2 : Gain  Gain=0.2
  Gain3 : Gain  Gain=0.1
  Gain4 : Gain  Gain=-0.5
  Gain5 : Gain  Gain=-10
  Gain6 : Gain  Gain=1.5
  Gain8 : Gain  Gain=-0.1
  Gain9 : Gain  Gain=-0.125
  Math Function2 : Math  Operator=square  SignedPower=on
  Square{1..4} (4 alike) : Math  Operator=square  SignedPower=on
  Sum1 : Sum  Inputs=+++++
  Unit Delay : UnitDelay  SampleTime=-1  HasFrameUpgradeWarning=on
  Unit Delay1 : UnitDelay  SampleTime=-1  HasFrameUpgradeWarning=on
  r_pf : Outport  VectorParamsAs1DForOutWhenUnconnected=off
  wires:
  Gain12/1 -> Sum1/1
  Gain6/1 -> Sum1/2
  Gain1/1 -> Sum1/3
  Gain2/1 -> Sum1/4
  Gain3/1 -> Sum1/5
  Exp4/1 -> Gain3/1
  Exp3/1 -> Gain2/1
  Exp2/1 -> Gain1/1
  Exp1/1 -> Gain6/1
  Gain9/1 -> Exp1/1
  Gain4/1 -> Exp2/1
  Gain5/1 -> Exp3/1
  Gain8/1 -> Exp4/1
  Square1/1 -> Gain9/1
  Math Function2/1 -> Gain5/1
  Square3/1 -> Gain8/1
  Unit Delay1/1 -> Square3/1
  Unit Delay/1 -> Math Function2/1  "u_prev"
  e2/1 -> Square2/1
  e1/1 -> Square1/1
  steer/1 -> Unit Delay/1
  Square2/1 -> Gain4/1
  accel/1 -> Unit Delay1/1
  Sum1/1 -> r_pf/1
  v_err/1 -> Square4/1
  Exp/1 -> Gain12/1
  Square4/1 -> Gain11/1
  Gain11/1 -> Exp/1

== system rewardLibrary/Obs // Reward 6-2/Subsystem ==
  v_ego : Inport
  v_ref : Inport  Port=2
  e1 : Inport  Port=3
  e2 : Inport  Port=4
  e1dot : Inport  Port=5
  e2dot : Inport  Port=6
  v_lead : Inport  Port=7
  xgap : Inport  Port=8
  ygap : Inport  Port=9
  Add : Sum  Inputs=+-
  Discrete-Time Integrator1 : DiscreteIntegrator  SampleTime=-1  ICPrevOutput=DiscIntNeverNeededParam  ICPrevScaledInput=DiscIntNeverNeededParam
  Discrete-Time Integrator2 : DiscreteIntegrator  SampleTime=-1  ICPrevOutput=DiscIntNeverNeededParam  ICPrevScaledInput=DiscIntNeverNeededParam
  Discrete-Time Integrator3 : DiscreteIntegrator  SampleTime=-1  ICPrevOutput=DiscIntNeverNeededParam  ICPrevScaledInput=DiscIntNeverNeededParam
  Lateral deviation : Scope
  Mux : Mux  Inputs=12
  obs : Outport  VectorParamsAs1DForOutWhenUnconnected=off
  v_err : Outport  Port=2  VectorParamsAs1DForOutWhenUnconnected=off
  wires:
  v_ref/1 -> Add/1  "d_rel"
  e2dot/1 -> Mux/9
  e1dot/1 -> Mux/8
  Mux/1 -> obs/1
  Discrete-Time Integrator2/1 -> Mux/4  "integral_error"
  e2/1 -> Discrete-Time Integrator3/1, Mux/7
  Discrete-Time Integrator1/1 -> Mux/1  "integral_error"
  e1/1 -> Discrete-Time Integrator2/1, Mux/5, Lateral deviation/1
  v_ego/1 -> Mux/3, Add/2
  Discrete-Time Integrator3/1 -> Mux/6  "integral_error"
  Add/1 -> Discrete-Time Integrator1/1, Mux/2, v_err/1
  v_lead/1 -> Mux/10
  xgap/1 -> Mux/11
  ygap/1 -> Mux/12

== system rewardLibrary/Obs // Reward 6-2/Subsystem2 ==
  v_ego : Inport
  e1 : Inport  Port=2
  e2 : Inport  Port=3
  xgap : Inport  Port=4
  collided : Inport  Port=5
  AND : Logic  IconShape=distinctive  AllPortsSameDT=off  OutDataTypeStr=boolean
  AND1 : Logic  IconShape=distinctive  AllPortsSameDT=off  OutDataTypeStr=boolean
  Abs : Abs  SaturateOnIntegerOverflow=off
  Abs1 : Abs  SaturateOnIntegerOverflow=off
  Compare To Constant : simulink/Logic and Bit Operations/Compare To Constant  relop=>  const=90  OutDataTypeStr=boolean
  Compare To Constant1 : simulink/Logic and Bit Operations/Compare To Constant  relop=>  const=0  OutDataTypeStr=boolean
  Constant : Constant
  Constant3 : Constant  Value=0
  Demux : Demux  Outputs=2
  Detect Rise Positive : simulink/Logic and Bit Operations/Detect Rise Positive  vinit=0  OutDataTypeStr=boolean
  Lateral deviation : simulink/Logic and Bit Operations/Compare To Constant  relop=>  const=8  OutDataTypeStr=boolean
  Logical Operator1 : Logic  Operator=OR  Inputs=3  AllPortsSameDT=off  OutDataTypeStr=boolean
  R2D : Gain  Gain=180/pi
  Relative yaw angle : simulink/Logic and Bit Operations/Compare To Constant  relop=>  const=55  OutDataTypeStr=boolean
  Switch : Switch  Criteria=u2 > Threshold  Threshold=90  SaturateOnIntegerOverflow=off  InputSameDT=off
  Terminator : Terminator
  Velocity : simulink/Logic and Bit Operations/Compare To Constant  relop=<  const=2  OutDataTypeStr=boolean
  Velocity1 : simulink/Logic and Bit Operations/Compare To Constant  relop=<  const=10  OutDataTypeStr=boolean
  fail : Outport  VectorParamsAs1DForOutWhenUnconnected=off
  failCollided : Outport  Port=2  VectorParamsAs1DForOutWhenUnconnected=off
  completeCourse : Outport  Port=3  VectorParamsAs1DForOutWhenUnconnected=off
  overtakeSuccess : Outport  Port=4  VectorParamsAs1DForOutWhenUnconnected=off
  wires:
  Demux/2 -> Compare To Constant/1, Switch/2  "y2"
  [pos2] -> Demux/1
  Demux/1 -> Terminator/1
  Logical Operator1/1 -> fail/1
  Constant3/1 -> Switch/3
  Constant/1 -> Switch/1
  Switch/1 -> completeCourse/1
  AND/1 -> Logical Operator1/3  "spinTurn"
  Relative yaw angle/1 -> AND/2
  R2D/1 -> Relative yaw angle/1
  Abs1/1 -> R2D/1
  e2/1 -> Abs1/1
  Velocity1/1 -> AND/1
  e1/1 -> Abs/1
  Abs/1 -> Lateral deviation/1
  v_ego/1 -> Velocity/1, Velocity1/1
  Lateral deviation/1 -> Logical Operator1/2
  Velocity/1 -> Logical Operator1/1  "tooSlow"
  Compare To Constant/1 -> Detect Rise Positive/1
  Detect Rise Positive/1 -> AND1/1
  xgap/1 -> Compare To Constant1/1
  Compare To Constant1/1 -> AND1/2
  AND1/1 -> overtakeSuccess/1
  collided/1 -> failCollided/1

== system rewardLibrary/Obs // Reward 6-3/Subsystem ==
  v_ego : Inport
  v_ref : Inport  Port=2
  e1 : Inport  Port=3
  e2 : Inport  Port=4
  e1dot : Inport  Port=5
  e2dot : Inport  Port=6
  v_lead : Inport  Port=7
  xgap : Inport  Port=8
  ygap : Inport  Port=9
  Add : Sum  Inputs=+-
  Discrete-Time Integrator1 : DiscreteIntegrator  SampleTime=-1  ICPrevOutput=DiscIntNeverNeededParam  ICPrevScaledInput=DiscIntNeverNeededParam
  Discrete-Time Integrator2 : DiscreteIntegrator  SampleTime=-1  ICPrevOutput=DiscIntNeverNeededParam  ICPrevScaledInput=DiscIntNeverNeededParam
  Discrete-Time Integrator3 : DiscreteIntegrator  SampleTime=-1  ICPrevOutput=DiscIntNeverNeededParam  ICPrevScaledInput=DiscIntNeverNeededParam
  Lateral deviation : Scope
  Mux : Mux  Inputs=12
  obs : Outport  VectorParamsAs1DForOutWhenUnconnected=off
  v_err : Outport  Port=2  VectorParamsAs1DForOutWhenUnconnected=off
  wires:
  v_ref/1 -> Add/1  "d_rel"
  e2dot/1 -> Mux/9
  e1dot/1 -> Mux/8
  Mux/1 -> obs/1
  Discrete-Time Integrator2/1 -> Mux/4  "integral_error"
  e2/1 -> Discrete-Time Integrator3/1, Mux/7
  Discrete-Time Integrator1/1 -> Mux/1  "integral_error"
  e1/1 -> Discrete-Time Integrator2/1, Mux/5, Lateral deviation/1
  v_ego/1 -> Mux/3, Add/2
  Discrete-Time Integrator3/1 -> Mux/6  "integral_error"
  Add/1 -> Discrete-Time Integrator1/1, Mux/2, v_err/1
  v_lead/1 -> Mux/10
  xgap/1 -> Mux/11
  ygap/1 -> Mux/12

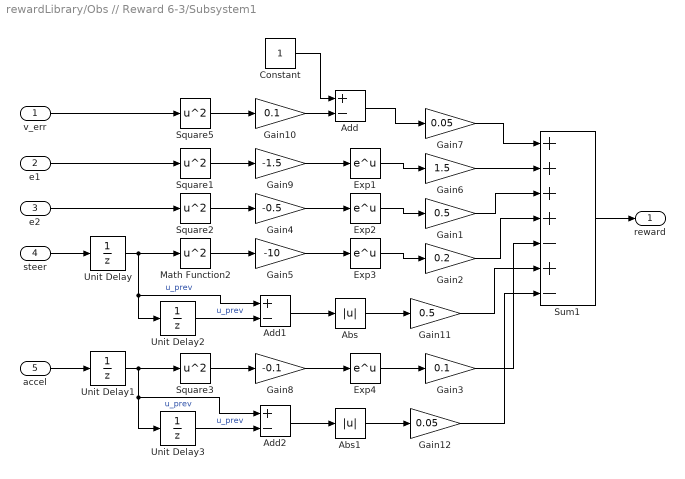
== system rewardLibrary/Obs // Reward 6-3/Subsystem1 ==
  v_err : Inport
  e1 : Inport  Port=2
  e2 : Inport  Port=3
  steer : Inport  Port=4
  accel : Inport  Port=5
  Abs : Abs  SaturateOnIntegerOverflow=off
  Abs1 : Abs  SaturateOnIntegerOverflow=off
  Add : Sum  Inputs=+-
  Add1 : Sum  Inputs=+-
  Add2 : Sum  Inputs=+-
  Constant : Constant
  Exp{1..4} (4 alike) : Math
  Gain1 : Gain  Gain=0.5
  Gain10 : Gain  Gain=0.1
  Gain11 : Gain  Gain=0.5
  Gain12 : Gain  Gain=0.05
  Gain2 : Gain  Gain=0.2
  Gain3 : Gain  Gain=0.1
  Gain4 : Gain  Gain=-0.5
  Gain5 : Gain  Gain=-10
  Gain6 : Gain  Gain=1.5
  Gain7 : Gain  Gain=0.05
  Gain8 : Gain  Gain=-0.1
  Gain9 : Gain  Gain=-1.5
  Math Function2 : Math  Operator=square  SignedPower=on
  Square{1..3,5} (4 alike) : Math  Operator=square  SignedPower=on
  Sum1 : Sum  Inputs=++++-+-
  Unit Delay{,1..3} (4 alike) : UnitDelay  SampleTime=-1  HasFrameUpgradeWarning=on
  reward : Outport  VectorParamsAs1DForOutWhenUnconnected=off
  wires:
  Gain10/1 -> Add/2
  Constant/1 -> Add/1
  Gain7/1 -> Sum1/1
  Gain6/1 -> Sum1/2
  Gain1/1 -> Sum1/3
  Gain2/1 -> Sum1/4
  Gain3/1 -> Sum1/5
  Exp4/1 -> Gain3/1
  Exp3/1 -> Gain2/1
  Exp2/1 -> Gain1/1
  Exp1/1 -> Gain6/1
  Add/1 -> Gain7/1
  Gain9/1 -> Exp1/1
  Gain4/1 -> Exp2/1
  Gain5/1 -> Exp3/1
  Gain8/1 -> Exp4/1
  Square1/1 -> Gain9/1
  Math Function2/1 -> Gain5/1
  Square3/1 -> Gain8/1
  e2/1 -> Square2/1
  v_err/1 -> Square5/1
  e1/1 -> Square1/1
  Square5/1 -> Gain10/1
  steer/1 -> Unit Delay/1
  Square2/1 -> Gain4/1
  accel/1 -> Unit Delay1/1
  Sum1/1 -> reward/1
  Abs/1 -> Gain11/1
  Unit Delay2/1 -> Add1/2  "u_prev"
  Add1/1 -> Abs/1
  Unit Delay/1 -> Unit Delay2/1, Add1/1, Math Function2/1  "u_prev"
  Gain11/1 -> Sum1/6
  Unit Delay1/1 -> Unit Delay3/1, Add2/1, Square3/1  "u_prev"
  Abs1/1 -> Gain12/1
  Add2/1 -> Abs1/1
  Unit Delay3/1 -> Add2/2  "u_prev"
  Gain12/1 -> Sum1/7

== system rewardLibrary/Obs // Reward 6-3/Subsystem2 ==
  v_ego : Inport
  e1 : Inport  Port=2
  e2 : Inport  Port=3
  AND : Logic  IconShape=distinctive  AllPortsSameDT=off  OutDataTypeStr=boolean
  Abs : Abs  SaturateOnIntegerOverflow=off
  Abs1 : Abs  SaturateOnIntegerOverflow=off
  Constant : Constant
  Constant3 : Constant  Value=0
  Demux : Demux  Outputs=2
  Lateral deviation : simulink/Logic and Bit Operations/Compare To Constant  relop=>  const=8  OutDataTypeStr=boolean
  Logical Operator1 : Logic  Operator=OR  AllPortsSameDT=off  OutDataTypeStr=boolean
  R2D : Gain  Gain=180/pi
  Relative yaw angle : simulink/Logic and Bit Operations/Compare To Constant  relop=>  const=60  OutDataTypeStr=boolean
  Switch : Switch  Criteria=u2 > Threshold  Threshold=90  SaturateOnIntegerOverflow=off  InputSameDT=off
  Terminator : Terminator
  Velocity : simulink/Logic and Bit Operations/Compare To Constant  relop=<  const=2  OutDataTypeStr=boolean
  Velocity1 : simulink/Logic and Bit Operations/Compare To Constant  relop=<  const=10  OutDataTypeStr=boolean
  fail : Outport  VectorParamsAs1DForOutWhenUnconnected=off
  success : Outport  Port=2  VectorParamsAs1DForOutWhenUnconnected=off
  fail_spinTurn : Outport  Port=3  VectorParamsAs1DForOutWhenUnconnected=off
  wires:
  Demux/2 -> Switch/2  "y2"
  [pos2] -> Demux/1
  Demux/1 -> Terminator/1
  Logical Operator1/1 -> fail/1
  Constant3/1 -> Switch/3
  Constant/1 -> Switch/1
  Switch/1 -> success/1
  AND/1 -> fail_spinTurn/1  "spinTurn"
  Relative yaw angle/1 -> AND/2
  R2D/1 -> Relative yaw angle/1
  Abs1/1 -> R2D/1
  e2/1 -> Abs1/1
  Velocity1/1 -> AND/1
  e1/1 -> Abs/1
  Abs/1 -> Lateral deviation/1
  v_ego/1 -> Velocity/1, Velocity1/1
  Lateral deviation/1 -> Logical Operator1/2
  Velocity/1 -> Logical Operator1/1  "tooSlow"

== system rewardLibrary/Obs // Reward 6-4/Subsystem ==
  v_ego : Inport
  v_ref : Inport  Port=2
  e1 : Inport  Port=3
  e2 : Inport  Port=4
  e1dot : Inport  Port=5
  e2dot : Inport  Port=6
  v_lead : Inport  Port=7
  xgap : Inport  Port=8
  ygap : Inport  Port=9
  Add : Sum  Inputs=+-
  Discrete-Time Integrator1 : DiscreteIntegrator  SampleTime=-1  ICPrevOutput=DiscIntNeverNeededParam  ICPrevScaledInput=DiscIntNeverNeededParam
  Discrete-Time Integrator2 : DiscreteIntegrator  SampleTime=-1  ICPrevOutput=DiscIntNeverNeededParam  ICPrevScaledInput=DiscIntNeverNeededParam
  Discrete-Time Integrator3 : DiscreteIntegrator  SampleTime=-1  ICPrevOutput=DiscIntNeverNeededParam  ICPrevScaledInput=DiscIntNeverNeededParam
  Lateral deviation : Scope
  Mux : Mux  Inputs=12
  obs : Outport  VectorParamsAs1DForOutWhenUnconnected=off
  v_err : Outport  Port=2  VectorParamsAs1DForOutWhenUnconnected=off
  wires:
  v_ref/1 -> Add/1  "d_rel"
  e2dot/1 -> Mux/9
  e1dot/1 -> Mux/8
  Mux/1 -> obs/1
  Discrete-Time Integrator2/1 -> Mux/4  "integral_error"
  e2/1 -> Discrete-Time Integrator3/1, Mux/7
  Discrete-Time Integrator1/1 -> Mux/1  "integral_error"
  e1/1 -> Discrete-Time Integrator2/1, Mux/5, Lateral deviation/1
  v_ego/1 -> Mux/3, Add/2
  Discrete-Time Integrator3/1 -> Mux/6  "integral_error"
  Add/1 -> Discrete-Time Integrator1/1, Mux/2, v_err/1
  v_lead/1 -> Mux/10
  xgap/1 -> Mux/11
  ygap/1 -> Mux/12
